simulink model "DCMotor_controlsim_older"  (R2024b)
settings: Solver=ode45  StartTime=0.0  StopTime=10  FixedStep=Ts  RelTol=1e-3
values from neighbouring files (symbols this model uses):
  alpha_F = 0.0002844    [Motor_control_script.m]
  J = 7.2e-3    (= 0.0072)    [Motor_control_script.m]
  Kawi = Kri    (= 1.56)    [Motor_control_script.m]
  Kawn = 50*Krn    (= 6.375)    [Motor_control_script.m]
  kG = 0.126    [Motor_control_script.m]
  Kri = LA/(2*Tfi + Ts)    (= 1.56)    [Motor_control_script.m]
  Krn = 0.1275    [Motor_control_script.m]
  La = LA    (= 0.0078)    [Motor_control_script.m]
  Ra = RA    (= 1.57)    [Motor_control_script.m]
  tau_F0 = 0.04631    [Motor_control_script.m]
  Tii = T1    (= 0.00496815286624)    [Motor_control_script.m]
  Tin = 1/11.03    (= 0.090661831369)    [Motor_control_script.m]
libraries: cstblocks x2
Description:
  | Water Tank Model with Dashboard
  | 
  | The example model "sldrtex_dashboard" shows a real-time model of a water tank
  | controlled by dashboard controls.  You can change the inputs to the plant using
  | the knobs and observe the response on the gauges.
  | 
  | How to run this model in Normal Mode:
  | 
  | 1) Double-click the orange button to switch to Normal Mode if needed.
  | 2) Start the real-time execution using Simulation->Run.
  | 3) Change the input flow and output valve values by the dashboard controls and observe
  |    the results on the dashboard gauges.
  | 
  | How to run this model in External Mode:
  | 
  | 1) Double-click the orange button to switch to External Mode if needed.
  | 2) Start the real-time execution using Simulation->Run. The model will automatically
  |    build, connect to Simulink in External Mode and start.
  | 3) Change the input flow and output valve values by the dashboard controls and observe
  |    the results on the dashboard gauges.
settings Model: SimulationMode=external  ExtModeTrigDuration=100001  Creator=The MathWorks, Inc.  LastModifiedBy=lenovo x390
settings SolverCC: AlgebraicLoopSolver=TrustRegion  AutoInsertRateTranBlk=on
settings DataIOCC: LimitDataPoints=on  SaveFormat=Array  ReturnWorkspaceOutputs=off  SignalLoggingName=logsOut
settings OptimizationCC: ExpressionDepthLimit=2147483647  InitFltsAndDblsToZero=on  EfficientMapNaN2IntZero=off  LifeSpan=inf
settings DebuggingCC: UnderspecifiedInitializationDetection=Classic  MergeDetectMultiDrivingBlocksExec=none  SignalResolutionControl=TryResolveAllWithWarning  FcnCallInpInsideContextMsg=warning  UnconnectedInputMsg=warning  UnconnectedOutputMsg=warning  UnconnectedLineMsg=warning  AllowSymbolicDim=off  StateNameClashWarn=warning  SFUnexpectedBacktrackingDiag=warning  SFNoUnconditionalDefaultTransitionDiag=warning  SFExecutionAtInitializationDiag=none  ArithmeticOperatorsInVariantConditions=warning
settings HardwareCC: ProdBitPerLong=64  ProdHWDeviceType=Intel->x86-64 (Linux 64)  TargetBitPerLong=64  TargetBitPerPointer=64  TargetBitPerSizeT=64  TargetBitPerPtrDiffT=64  TargetIntDivRoundTo=Zero  TargetEndianess=LittleEndian  TargetWordSize=64  TargetHWDeviceType=Intel->x86-64
settings ModelReferenceCC: EnableRefExpFcnMdlSchedulingChecks=on  PropagateSignalLabelsOutOfModel=off
settings SFSimCC: SimUseLocalCustomCode=off  CustomCodeUndefinedFunction=UseInterfaceOnly
settings RTWCC: Description=Simulink Desktop Real-Time  SystemTargetFile=sldrt.tlc  TemplateMakefile=sldrt.tmf  RTWUseLocalCustomCode=off  RTWCompilerOptimization=on  GPUComputeCapability=3.5  DLArmComputeVersion=19.05
settings CodeAppCC: MaxIdLength=95  StateflowObjectComments=on
settings SimulinkDesktopRealTimeCC: TargetLibSuffix=_sldrt.a  TargetPreCompLibLocation=C:\Program Files\MATLAB\R2024A\toolbox\sldrt\lib\win64  SupportVariableSizeSignals=off
settings ConfigComp: CovMetricSettings=dw  CovSaveCumulativeToWorkspaceVar=on  CovSaveSingleToWorkspaceVar=on  CovExternalEMLEnable=off  CovSFcnEnable=off

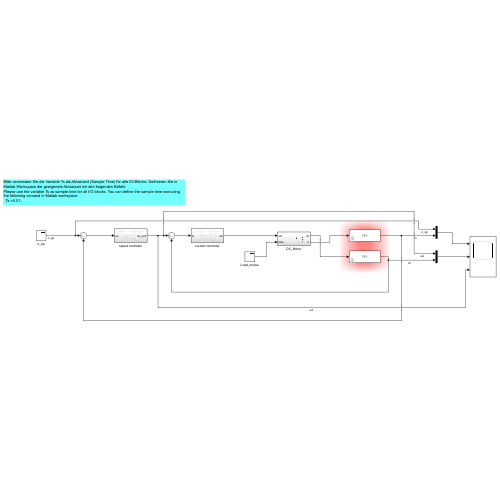
[thumbnail: Simulink's stored preview of the top-level diagram]
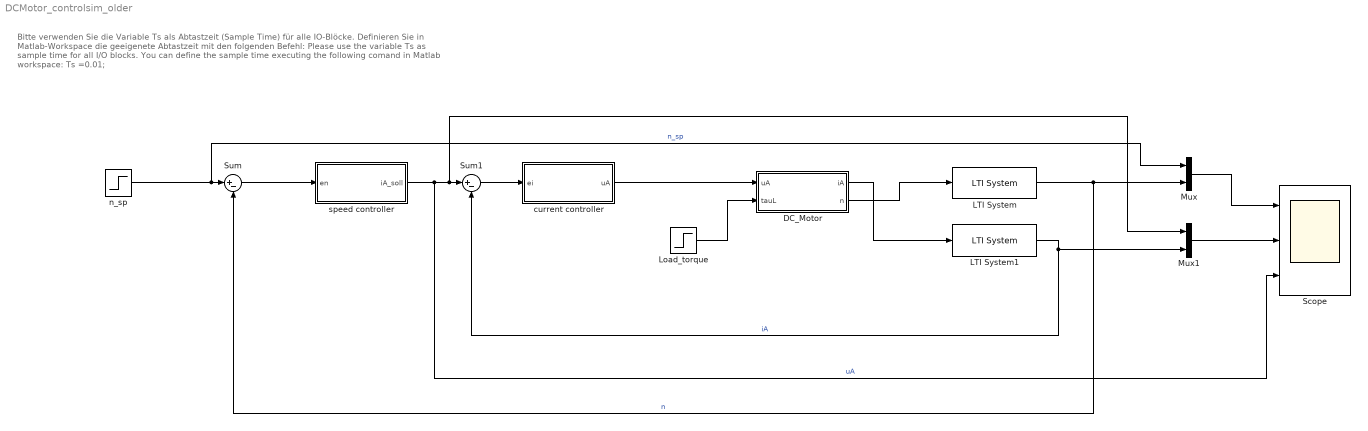
== system DCMotor_controlsim_older ==
  note: Bitte verwenden Sie die Variable Ts als Abtastzeit (Sample Time) für alle IO-Blöcke. Definieren Sie in Matlab-Workspace die geeigenete Abtastzeit mit den folgenden Befehl:
      | Please use the variable Ts as sample time for all I/O blocks. You can define the sample time executing the following comand in Matlab workspace:
      |   Ts =0.01;
  DC_Motor : Subsystem
  LTI System : cstblocks/LTI System  sys=Gfn  IC=[]  PadeOrder=0
  LTI System1 : cstblocks/LTI System  sys=Gfi  IC=[]  PadeOrder=0
  Load_torque : Step  Time=6  After=0.3  SampleTime=0
  Mux : Mux  Inputs=2
  Mux1 : Mux  Inputs=2
  Scope : Scope  NumInputPorts=3
  Sum : Sum  Inputs=|+-
  Sum1 : Sum  Inputs=|+-
  current controller : Subsystem
  n_sp : Step  After=2000  SampleTime=0
  speed controller : Subsystem
  wires:
  n_sp/1 -> Mux/1, Sum/1  "n_sp"
  Sum/1 -> speed controller/1(en)
  speed controller/1(iA_soll) -> Scope/3, Mux1/1, Sum1/1  "uA"
  Sum1/1 -> current controller/1(ei)
  current controller/1(uA) -> DC_Motor/1(uA)
  Load_torque/1 -> DC_Motor/2(tauL)
  LTI System1/1 -> Mux1/2, Sum1/2  "iA"
  LTI System/1 -> Mux/2, Sum/2  "n"
  Mux/1 -> Scope/1
  Mux1/1 -> Scope/2
  DC_Motor/2(n) -> LTI System/1
  DC_Motor/1(iA) -> LTI System1/1

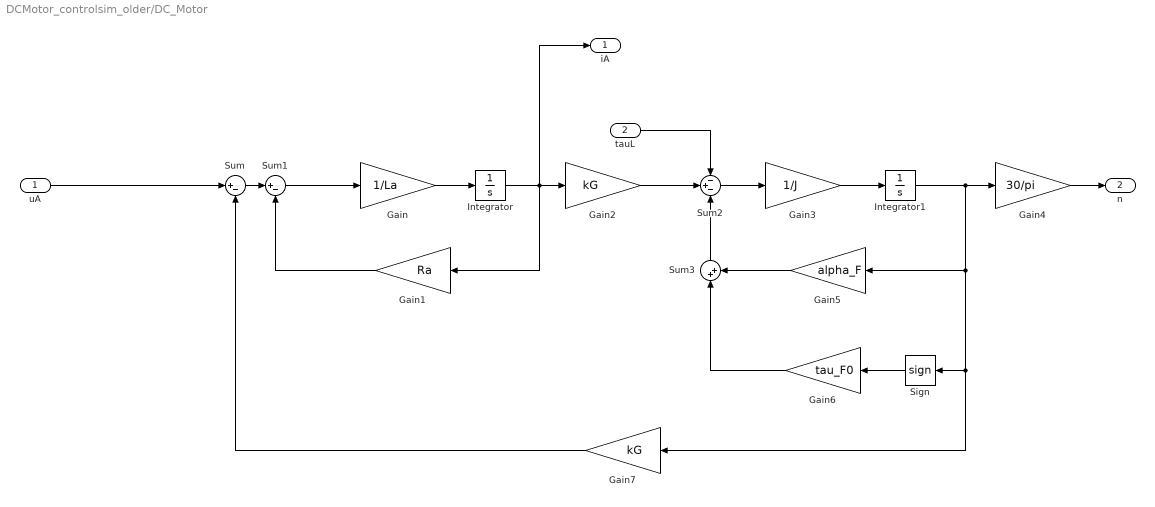
== system DCMotor_controlsim_older/DC_Motor ==
  uA : Inport
  tauL : Inport  Port=2
  Gain : Gain  Gain=1/La
  Gain1 : Gain  Gain=Ra
  Gain2 : Gain  Gain=kG
  Gain3 : Gain  Gain=1/J
  Gain4 : Gain  Gain=30/pi
  Gain5 : Gain  Gain=alpha_F
  Gain6 : Gain  Gain=tau_F0
  Gain7 : Gain  Gain=kG
  Integrator : Integrator
  Integrator1 : Integrator
  Sign : Signum
  Sum : Sum  Inputs=|+-
  Sum1 : Sum  Inputs=|+-
  Sum2 : Sum  Inputs=-+-
  Sum3 : Sum  Inputs=|++
  iA : Outport
  n : Outport  Port=2
  wires:
  uA/1 -> Sum/1
  Gain/1 -> Integrator/1
  Integrator/1 -> iA/1, Gain1/1, Gain2/1
  Sum/1 -> Sum1/1
  Sum1/1 -> Gain/1
  Gain1/1 -> Sum1/2
  Gain2/1 -> Sum2/2
  tauL/1 -> Sum2/1
  Gain3/1 -> Integrator1/1
  Integrator1/1 -> Sign/1, Gain7/1, Gain5/1, Gain4/1
  Gain4/1 -> n/1
  Sum2/1 -> Gain3/1
  Sum3/1 -> Sum2/3
  Gain5/1 -> Sum3/2
  Gain6/1 -> Sum3/1
  Sign/1 -> Gain6/1
  Gain7/1 -> Sum/2

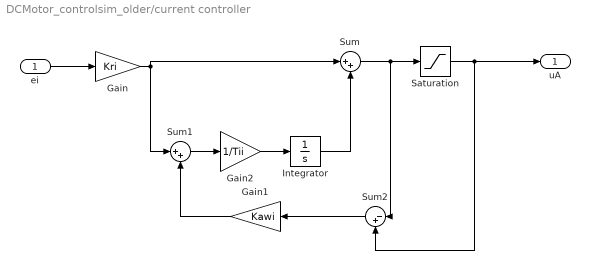
== system DCMotor_controlsim_older/current controller ==
  ei : Inport
  Gain : Gain  Gain=Kri
  Gain1 : Gain  Gain=Kawi
  Gain2 : Gain  Gain=1/Tii
  Integrator : Integrator
  Saturation : Saturate  UpperLimit=42  LowerLimit=-42
  Sum : Sum  Inputs=|++
  Sum1 : Sum  Inputs=|++
  Sum2 : Sum  Inputs=|-+
  uA : Outport
  wires:
  Integrator/1 -> Sum/2
  Gain/1 -> Sum/1, Sum1/1
  Sum/1 -> Saturation/1, Sum2/1
  Sum1/1 -> Gain2/1
  Saturation/1 -> uA/1, Sum2/2
  Gain1/1 -> Sum1/2
  Sum2/1 -> Gain1/1
  Gain2/1 -> Integrator/1
  ei/1 -> Gain/1

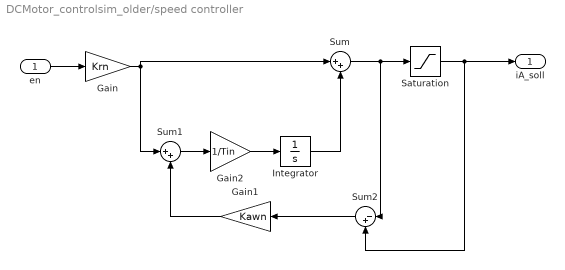
== system DCMotor_controlsim_older/speed controller ==
  en : Inport
  Gain : Gain  Gain=Krn
  Gain1 : Gain  Gain=Kawn
  Gain2 : Gain  Gain=1/Tin
  Integrator : Integrator
  Saturation : Saturate  UpperLimit=10  LowerLimit=-10
  Sum : Sum  Inputs=|++
  Sum1 : Sum  Inputs=|++
  Sum2 : Sum  Inputs=|-+
  iA_soll : Outport
  wires:
  en/1 -> Gain/1
  Gain/1 -> Sum/1, Sum1/1
  Sum1/1 -> Gain2/1
  Gain2/1 -> Integrator/1
  Integrator/1 -> Sum/2
  Gain1/1 -> Sum1/2
  Sum2/1 -> Gain1/1
  Sum/1 -> Saturation/1, Sum2/1
  Saturation/1 -> iA_soll/1, Sum2/2
